simulink model "webcam_test"  (Simulink 7.8)
settings: Solver=ode45  StartTime=0.0  StopTime=10.0  RelTol=1e-3
undefined symbols (not defined in the file): gray, jet, none, videoinput
libraries: visionsinks x3, imaqlib x1
settings Model: Creator=wildcat  LastModifiedBy=wildcat

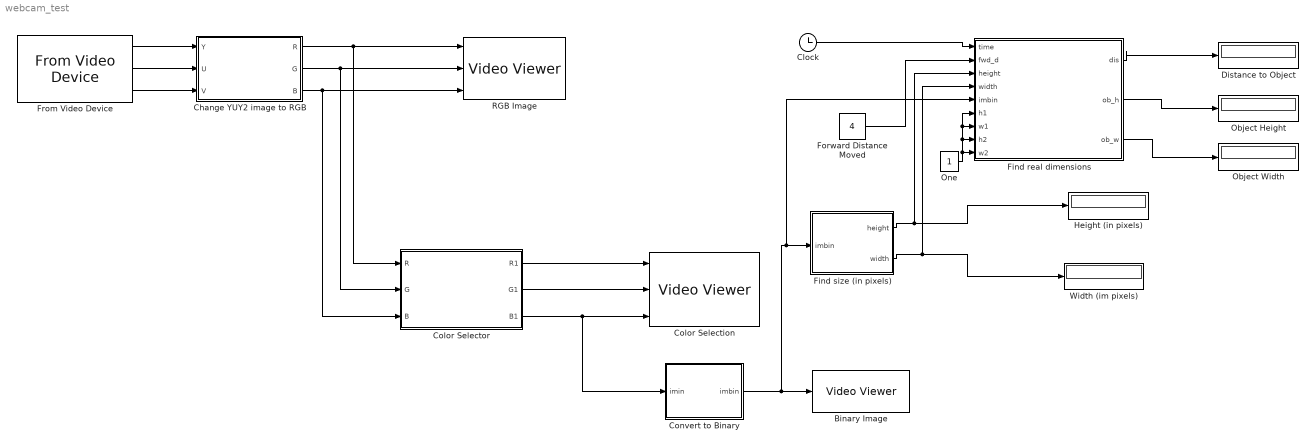
== system webcam_test ==
  Binary Image : visionsinks/Video Viewer  inputType=Obsolete7b  imagePorts=One multidimensional signal  useColorMap=off  colormapValue=jet(256)  specRange=off  minInputVal=0  maxInputVal=255  FigPos=[482 533 406 310]  AxisZoom=on  trueSizedOnce=off  OpenAtMdlStart=on
  Change YUY2 image to RGB : MATLAB Function  TreatAsAtomicUnit=on
  Clock : Clock
      settings: Decimation=30
  Color Selection : visionsinks/Video Viewer  inputType=Obsolete7b  imagePorts=Separate color signals  useColorMap=off  colormapValue=gray(256)  specRange=off  minInputVal=0  maxInputVal=255  FigPos=[67 663 787 535]  AxisZoom=on  trueSizedOnce=off  OpenAtMdlStart=on
  Color Selector : MATLAB Function  TreatAsAtomicUnit=on
  Convert to Binary : MATLAB Function  TreatAsAtomicUnit=on
  Distance to Object : Display
  Find real dimensions : MATLAB Function  TreatAsAtomicUnit=on
  Find size (in pixels) : MATLAB Function  TreatAsAtomicUnit=on
  Forward Distance Moved : Constant  Value=4
  From Video Device : imaqlib/From Video Device  DeviceMenu=winvideo 1 (Microsoft LifeCam HD-3000)  Device=winvideo 1 (Microsoft LifeCam HD-3000)  ObjConstructor=videoinput('winvideo', 1)  VideoFormatMenu=YUY2_640x480  VideoFormat=YUY2_640x480  VideoSource=input1  ROIPosition=[0 0 480 640]  EnableHWTrigger=off  TriggerConfiguration=none/none  SampleTime=1/30  OutputPortsMode=Separate color signals  DataType=uint8  CanDoHWTrigger=no  ReturnedColorSpace=YCbCr  BlockHandle=1973.0006  ROIWidth=640  ROIHeight=480  ROIColumn=0  ROIRow=0  EngXMLPath=C:\Program Files\MatlabR2011b\toolbox\imaq\imaq\private  DevXMLPath=C:\Program Files\MatlabR2011b\toolbox\imaq\imaqadaptors\win64  EngLibPath=C:\Program Files\MatlabR2011b\toolbox\imaq\imaqblks\imaqmex\win64
  Height (in pixels) : Display
  Object Height : Display
  Object Width : Display
  One : Constant
  RGB Image : visionsinks/Video Viewer  inputType=Obsolete7b  imagePorts=Separate color signals  useColorMap=off  colormapValue=gray(256)  specRange=off  minInputVal=0  maxInputVal=255  FigPos=[175 685 640 500]  AxisZoom=on  trueSizedOnce=off  OpenAtMdlStart=on
  Width (im pixels) : Display
  wires:
  From Video Device/1 -> Change YUY2 image to RGB/1(Y)
  From Video Device/2 -> Change YUY2 image to RGB/2(U)
  From Video Device/3 -> Change YUY2 image to RGB/3(V)
  Change YUY2 image to RGB/3(B) -> Color Selector/3(B), RGB Image/3
  Change YUY2 image to RGB/2(G) -> Color Selector/2(G), RGB Image/2
  Change YUY2 image to RGB/1(R) -> Color Selector/1(R), RGB Image/1
  Color Selector/1(R1) -> Color Selection/1
  Color Selector/2(G1) -> Color Selection/2
  Color Selector/3(B1) -> Color Selection/3, Convert to Binary/1(imin)
  Convert to Binary/1(imbin) -> Binary Image/1, Find size (in pixels)/1(imbin), Find real dimensions/5(imbin)
  Find size (in pixels)/1(height) -> Height (in pixels)/1, Find real dimensions/3(height)
  Find size (in pixels)/2(width) -> Width (im pixels)/1, Find real dimensions/4(width)
  Forward Distance Moved/1 -> Find real dimensions/2(fwd_d)
  Find real dimensions/1(dis) -> Distance to Object/1
  Find real dimensions/2(ob_h) -> Object Height/1
  Find real dimensions/3(ob_w) -> Object Width/1
  Clock/1 -> Find real dimensions/1(time)
  One/1 -> Find real dimensions/6(h1), Find real dimensions/7(w1), Find real dimensions/8(h2), Find real dimensions/9(w2)

== matlab function Change YUY2 image to RGB ==
  data: Y input double; R output double; G output double; B output double; U input double; V input double
function [R,G,B] = YUY2toRGB(Y,U,V)
%% input is (:,:,1:3), where
%% (:,:,1) is Y, (:,:,2) is U, (:,:,3) is V


%Y = single(data(:,:,1));
%U = single(data(:,:,2));
%V = single(data(:,:,3));

B = 1.164*(Y - 16) + 2.018*(U - 128);

G = 1.164*(Y - 16) - 0.813*(V - 128) - 0.391*(U - 128);

R = 1.164*(Y - 16) + 1.596*(V - 128);

R=uint8(R);
G=uint8(G);
B=uint8(B);

== matlab function Color Selector ==
  data: R input double; R1 output double; G input double; B input double; G1 output double; B1 output double
function [R1,G1,B1] = color_selection(R,G,B)

imsize = size(R);
imsize = size(G);
imsize = size(B);

R1 = zeros(imsize);
G1 = zeros(imsize);
B1 = zeros(imsize);

for (imh = 1:imsize(1,1));
    for (iml = 1:imsize(1,2));
        imR = R(imh,iml);
        imG = G(imh,iml);
        imB = B(imh,iml);
        if (imR >= 245) && (imR <= 255) && (imG >= 115) && (imG <= 200) && (imB >= 165) && (imB <= 215)
            R1(imh,iml) = 255;
            G1(imh,iml) = 255;
            B1(imh,iml) = 255;
        end
    end
end

== matlab function Convert to Binary ==
  data: imin input double; imbin output double
function imbin = bin_conv(imin)

imsize = size(imin);
imbin=zeros(imsize);

for (imh = 1:imsize(1,1));
    for (iml = 1:imsize(1,2));
        imloc = imin(imh,iml);
        if (imloc == 255)
            imbin(imh,iml) = 1;
        end
    end
end

== matlab function Find size (in pixels) ==
  data: imbin input double; height output double; width output double
function [height,width] = hw_find(imbin)

imsize=size(imbin);

height = 0;
width = 0;
height_sum = 0;
width_sum = 0;

for (imh = 1:imsize(1,1));
    width_sum;
    for (iml = 1:imsize(1,2));
        imloc = imbin(imh,iml);
        if (imloc == 1)
            width_sum=width_sum+1;
        end
    end
    if (width_sum >= 50)
        height = height+1;
    end
end

for (iml = 1:imsize(1,2));
    height_sum = 0;
    for (imh = 1:imsize(1,1));
        imloc = imbin(imh,iml);
        if (imloc == 1)
            height_sum=height_sum+1;
        end
    end
    if (height_sum >= 30)
        width = width+1;
    end
end

== matlab function Find real dimensions ==
  data: time input double; dis output double; fwd_d input double; height input double; width input double; ob_h output double; ob_w output double; imbin input double; h1 input double; w1 input double; h2 input double; w2 input double
function [dis,ob_h,ob_w] = real_dim_find(time,fwd_d,height,width,imbin,h1,w1,h2,w2)

size1 = size(imbin);
hsample = height;
wsample = width;

if (time <= 1)
    h1=1;
    h2=2;
elseif (time == 1)
    h1=height;
    w1=width;
else
    h1=h1;
    w1=w1;
end


if (time <= 3)
    h1=1;
    w2=2;
elseif (time == 3)
    h2=height;
    w2=width;
else
    h2=h2;
    w2=w2;
end

ratio1=h2/h1;
dis=(fwd_d*ratio1)/(ratio1-1);
ob_h=2*tan(44.443*pi/360)*dis*h1/size1(1,1);
ob_w=2*tan(57.154*pi/360)*dis*w1/size1(1,2);
